simulink model "test_ball"  (R2019b)
settings: Solver=VariableStepAuto  StartTime=0.0  StopTime=10.0  RelTol=1e-3
settings Model: Creator=patate  LastModifiedBy=patate

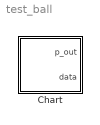
== system test_ball ==
  Chart : Stateflow chart  BlockKeywords=__PRM__SERIALIZED__DATA__:Stateflow Chart,Stateflow Diagram  TreatAsAtomicUnit=on

== stateflow chart test_ball/Chart ==
  settings: updateMethod=CONTINUOUS
  state Name
    x=0;
  (default) -> Name : {
      | p = 10;
      | v = 15;
      | }
  data: v local double; p_out output double; p local double; data output double
  data v settings: updateMethod=SF_CONTINUOUS_TIME_DATA
  data p settings: updateMethod=SF_CONTINUOUS_TIME_DATA
